simulink model "aae564hw01syssoln"  (R2017b)
settings: Solver=VariableStepAuto  StartTime=0.0  StopTime=100.0  RelTol=1e-3
values from neighbouring files (symbols this model uses):
  l = [1 0.5]'    [aae564hw01soln.m]
  m = [2 1 1]'    [aae564hw01soln.m]    (also in aae564hw06.m; aae564hw08.m = [2 1 1]; aae564hw11.m = 0.5; aae564hw12.m = rand)
  q_0 = [0 -90.01 90]'    [aae564hw01soln.m]    (also in aae564hw06.m = x_0(1:3); aae564hw08.m = [y_e theta1_e theta2_e]')
  q_dot_0 = [0 0 0]'    [aae564hw01soln.m]    (also in aae564hw06.m = x_0(4:6); aae564hw08.m)
undefined symbols (not defined in the file or in its folder): get_q_ddot_double_pendulum
settings Model: Creator=mayer15  LastModifiedBy=mayer15

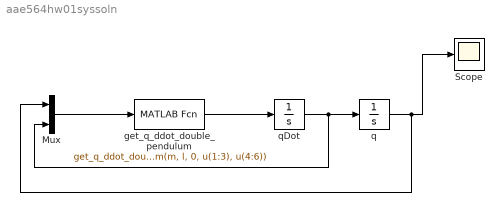
== system aae564hw01syssoln ==
  Mux : Mux  Inputs=2
  Scope : Scope
  get_q_ddot_double_pendulum : MATLABFcn  MATLABFcn=get_q_ddot_double_pendulum(m, l, 0, u(1:3), u(4:6))  OutputDimensions=3
  "q " : Integrator  InitialCondition=q_0
  "qDot " : Integrator  InitialCondition=q_dot_0
  wires:
  get_q_ddot_double_pendulum/1 -> "qDot "/1
  "qDot "/1 -> Mux/2, "q "/1
  "q "/1 -> Mux/1, Scope/1
  Mux/1 -> get_q_ddot_double_pendulum/1
